simulink library "LopesDevelopmentLibrary"  (R2015b)
settings: Solver=ode45  StartTime=0.0  StopTime=10.0  RelTol=1e-3
values from neighbouring files (symbols this model uses):
  d2r = @(d) d*(pi/180)    [LopesDevelopmentLibrary_LoadParameters.m]
  ts = LopesParams.ts    [LopesDevelopmentLibrary_LoadParameters.m]
undefined symbols (not defined in the file or in its folder): anyParameterChanged, DiscIntNeverNeededParam, gcbh, LHF, LKF, LopesParams, macaddr, mxpcnetworkconfig, mxpcrtudprx, mxpcrtudptx, patientParametersChanged, port, PX, PZ, RHF, RKF, SelectorLOPESInSize, StrideTime_s, Time
undefined symbols (not defined in the file): LopesParamsSendDataArrayLen
libraries: LopesDevelopmentLibrary x288, simulink x98, dspmtrx3 x47, xpciplib x6, xpcnetworkbufferlib x5, dspsigops x4, dspstat3 x3, xpcethernetlib x2, visionstatistics x2, xpcseriallib x2, nmc x1, simulink_extras x1
(part 8 of 12)

== system LopesDevelopmentLibrary/BlocksForInternalUse/LLC Communication/UDP_Blocks/Receive_RT_2015b ==
  Buffer 1 : xpcnetworkbufferlib/Manage   ChainSize=1  BufferSize=0  Threshold=0
  Extract 1 : xpcnetworkbufferlib/Extract   PacketSize=Receive3
  Terminator : Terminator
  UDP Consume 1 : xpciplib/UDP Consume   Group=udpID  VectorSize=0  SampleTime=Receive4
  UDP Rx 1 : xpciplib/UDP Rx   Priority=5  Group=udpID  sip=Any  SourceAddress=Receive1  lup=Specify  LocalPort=Receive2  SampleTime=Receive4
  Out1 : Outport  OutDataTypeStr=uint8
  Out2 : Outport  Port=2  OutDataTypeStr=double
  wires:
  UDP Consume 1/2 -> Terminator/1
  UDP Consume 1/1 -> Extract 1/1
  UDP Rx 1/1 -> Buffer 1/1
  Buffer 1/1 -> UDP Consume 1/1
  Extract 1/1 -> Out1/1
  Extract 1/2 -> Out2/1

== system LopesDevelopmentLibrary/BlocksForInternalUse/LLC Communication/UDP_Blocks/Send_RT_2012b ==
  In1 : Inport  OutDataTypeStr=uint8
  In2 : Inport  Port=2  OutDataTypeStr=double
  "Compose " : S-Function  FunctionName=xpcnbcompose  SFunctionDeploymentMode=off  EnableBusSupport=off  mask(xpcnbcompose){}
      mask help: Network Buffer Compose
      mask init:
      | mxpcnbcompose(2);
      mask Help: helpview(fullfile(docroot, 'mapfiles', 'xpc.map'), 'NB_Compose')
      mask Display: disp('NB Compose\n');port_label('input', 2, 'length');
  "UDP Produce " : S-Function  Priority=5  FunctionName=xpcudpproduce  Parameters=Group, SrcIp, sip, DstIp, dip, LocPort, lup, RemPort, rup, SampleTime  SFunctionDeploymentMode=off  EnableBusSupport=off  mask(udpproduce){Group=0, sip=Auto, SrcIp=0.0.0.0, dip=Specify, DstIp=Send1, rup=Specify, RemPort=Send2, lup=Auto, LocPort=Send3, SampleTime=Send4}
      mask prompts: Group "IP Group"; sip "Source IP Address"; SrcIp "Source IP Address"; dip "Destination IP Address"; DstIp "IP address to send to (255.255.255.255 for broadcast):"; rup "Remote UDP Port"; RemPort "Remote IP port to send to:"; lup "Local UDP Port"; LocPort "Use the following local IP port (-1 for automatic assignment):"; SampleTime "Sample time:"
      mask help: UDP Produce
      mask init:
      | if LocPort == -1
      |     lup = 3;
      | end
      | 
      | SrcIp = ipaddr(SrcIp);
      | DstIp = ipaddr(DstIp);
      mask Help: helpview(fullfile(docroot, 'mapfiles', 'xpc.map'), 'RT_UDP_PRODUCE')
      mask TypeOptions sip: Specify | Port | Auto
      mask TypeOptions dip: Specify | Port
      mask TypeOptions rup: Specify | Port
      mask TypeOptions lup: Specify | Port | Auto
      mask Display: disp('UDP Produce');
  "UDP Tx " : xpciplib/UDP Tx   Priority=5  Group=0  TTL=-1  ToS=-1  SampleTime=Send4
  wires:
  "UDP Produce "/1 -> "UDP Tx "/1
  "Compose "/1 -> "UDP Produce "/1
  In1/1 -> "Compose "/1
  In2/1 -> "Compose "/2

== system LopesDevelopmentLibrary/BlocksForInternalUse/LLC Communication/UDP_Blocks/Send_RT_2014b ==
  In1 : Inport  OutDataTypeStr=uint8
  In2 : Inport  Port=2  OutDataTypeStr=double
  "Compose " : S-Function  FunctionName=xpcnbcompose  SFunctionDeploymentMode=off  EnableBusSupport=off  mask(xpcnbcompose){}
      mask help: Network Buffer Compose
      mask init:
      | mxpcnbcompose(2);
      mask Help: helpview(fullfile(docroot, 'mapfiles', 'xpc.map'), 'NB_Compose')
      mask Display: disp('NB Compose\n');port_label('input', 2, 'length');
  "UDP Produce " : S-Function  Priority=5  FunctionName=xpcudpproduce  Parameters=Group, SrcIp, sip, DstIp, dip, LocPort, lup, RemPort, rup, SampleTime  SFunctionDeploymentMode=off  EnableBusSupport=off  mask(udpproduce){Group=udpID, sip=Auto, SrcIp=0.0.0.0, dip=Specify, DstIp=Send1, rup=Specify, RemPort=Send2, lup=Auto, LocPort=Send3, SampleTime=Send4}
      mask prompts: Group "IP Group"; sip "Source IP Address"; SrcIp "Source IP Address"; dip "Destination IP Address"; DstIp "IP address to send to (255.255.255.255 for broadcast):"; rup "Remote UDP Port"; RemPort "Remote IP port to send to:"; lup "Local UDP Port"; LocPort "Use the following local IP port (-1 for automatic assignment):"; SampleTime "Sample time:"
      mask help: UDP Produce
      mask init:
      | if LocPort == -1
      |     lup = 3;
      | else
      |     lup = 1;
      | end
      | 
      | SrcIp = ipaddr(SrcIp);
      | DstIp = ipaddr(DstIp);
      mask Help: helpview(fullfile(docroot, 'mapfiles', 'xpc.map'), 'RT_UDP_PRODUCE')
      mask TypeOptions sip: Specify | Port | Auto
      mask TypeOptions dip: Specify | Port
      mask TypeOptions rup: Specify | Port
      mask TypeOptions lup: Specify | Port | Auto
      mask Display: disp('UDP Produce');
  "UDP Tx " : xpciplib/UDP Tx   Priority=5  Group=udpID  TTL=-1  ToS=-1  SampleTime=Send4
  wires:
  "UDP Produce "/1 -> "UDP Tx "/1
  "Compose "/1 -> "UDP Produce "/1
  In1/1 -> "Compose "/1
  In2/1 -> "Compose "/2

== system LopesDevelopmentLibrary/BlocksForInternalUse/LLC Communication/UDP_Blocks/Send_RT_2015b ==
  In1 : Inport  OutDataTypeStr=uint8
  In2 : Inport  Port=2  OutDataTypeStr=double
  "Compose " : xpcnetworkbufferlib/Compose 
  "UDP Produce " : xpciplib/UDP Produce   Priority=5  Group=udpID  sip=Auto  SrcIp=0.0.0.0  dip=Specify  DstIp=Send1  rup=Specify  RemPort=Send2  lup=Auto  LocPort=Send3  SampleTime=Send4
  "UDP Tx " : xpciplib/UDP Tx   Priority=5  Group=udpID  TTL=-1  ToS=-1  SampleTime=Send4
  wires:
  "UDP Produce "/1 -> "UDP Tx "/1
  "Compose "/1 -> "UDP Produce "/1
  In1/1 -> "Compose "/1
  In2/1 -> "Compose "/2

== system LopesDevelopmentLibrary/GaitGeneration/CalculateBreaksCoefs/Calculate/ActuatedDOFS ==

== system LopesDevelopmentLibrary/GaitGeneration/CalculateBreaksCoefs/Calculate/GenerateFakeTime ==
  note: This block generates a 'fake time' signal: (a placeholder) and a
      | fake StrideTime. These are provided in order to be able to use block that
      | require the existence of these signals. By giving fake (i.e., wrong) values,
      | the calculations in those blocks involving these signals will be wrong, but these
      | calculations are never used, so this does not matter.
  Bus Creator13 : BusCreator  Inputs=2
  FakeBreaksTime : Constant  Value=[0,100]
  FakeCoefsTime : Constant  Value=[0,0,0;0,0,0]
  FakeStrideTime1 : Constant
  FakeStrideTime_s : Outport
  FakeTime : Outport  Port=2
  wires:
  FakeCoefsTime/1 -> Bus Creator13/2  "coefs"
  FakeBreaksTime/1 -> Bus Creator13/1  "breaks"
  Bus Creator13/1 -> FakeTime/1  "Time"
  FakeStrideTime1/1 -> FakeStrideTime_s/1

== system LopesDevelopmentLibrary/GaitGeneration/CalculateBreaksCoefs/Calculate/LeftAnkleZ1 ==
  note: Maximum of 15 cm extra circumduction
  parameters : Inport
  WeightShift_StepWidth_pct : Inport  Port=2
  Circumduction_CircumductionLeft_pct : Inport  Port=3
  AddToMatrixElement : LopesDevelopmentLibrary/Various/AddToMatrixElement  row=3  col=2  minimum=-inf  maximum=inf
  AssignMatrixElement : LopesDevelopmentLibrary/Various/AssignMatrixElement  row=3  col=2  minimum=-inf  maximum=inf
  Bias : Bias  Bias=1
  CircumductionGain : Gain  Gain=0.01*(-0.15)
  Gain2 : Gain  Gain=0.01
  K1toK3 : dspmtrx3/Submatrix  RowSpan=All rows  RowStartMode=Index  RowStartIndex=row  RowEndMode=Index  RowEndIndex=1  ColSpan=One column  ColStartMode=Index  ColStartIndex=2  ColEndMode=Last  ColEndIndex=1
  MinMax : MinMax
  MultiplyMatrixElement : LopesDevelopmentLibrary/Various/MultiplyMatrixElement  row=1  col=2  minimum=-inf  maximum=inf
  MultiplyMatrixElement1 : LopesDevelopmentLibrary/Various/MultiplyMatrixElement  row=2  col=2  minimum=-inf  maximum=inf
  RegressionData : Constant  Value=LopesParams.GaitData.LAnkleZ
  RegressionData2KeyEvents : LopesDevelopmentLibrary/BlocksForInternalUse/GaitGeneration/RegressionData2KeyEvents
  KeyEvents : Outport
  wires:
  RegressionData2KeyEvents/1 -> MultiplyMatrixElement/1
  RegressionData/1 -> RegressionData2KeyEvents/1
  parameters/1 -> RegressionData2KeyEvents/2
  WeightShift_StepWidth_pct/1 -> Gain2/1
  Gain2/1 -> Bias/1
  Bias/1 -> MultiplyMatrixElement/2, MultiplyMatrixElement1/2
  AddToMatrixElement/1 -> KeyEvents/1
  MultiplyMatrixElement/1 -> MultiplyMatrixElement1/1
  MultiplyMatrixElement1/1 -> K1toK3/1, AssignMatrixElement/1
  K1toK3/1 -> MinMax/1
  MinMax/1 -> AssignMatrixElement/2
  AssignMatrixElement/1 -> AddToMatrixElement/1
  Circumduction_CircumductionLeft_pct/1 -> CircumductionGain/1
  CircumductionGain/1 -> AddToMatrixElement/2

== system LopesDevelopmentLibrary/GaitGeneration/CalculateBreaksCoefs/Calculate/LeftHipFlexion1 ==
  parameters : Inport
  HipExtensionOffset_pct : Inport  Port=2
  Steplength_Length_pct : Inport  Port=3
  SteplengthOtherLeg_Length_pct : Inport  Port=4
  StepHeight_KneeFlexion_pct : Inport  Port=5
  AddToMatrixColumn : LopesDevelopmentLibrary/Various/AddToMatrixColumn  col=2  minimum=-inf  maximum=inf
  Bias : Bias  Bias=100
  Bias1 : Bias  Bias=100
  Gain1 : Gain  Gain=1/100
  Gain2 : Gain  Gain=1/100
  Gain3 : Gain  Gain=0.01* d2r(2.5)
  Gain4 : Gain  Gain=0.01* d2r(5)
  GainHipExtensionOffset : Gain  Gain=-0.01* d2r(10)
  KneeFlexionStepheight : LopesDevelopmentLibrary/Various/AddToMatrixElement  row=5  col=2  minimum=0  maximum=d2r(90)
  KneeFlexionStepheight1 : LopesDevelopmentLibrary/Various/AddToMatrixElement  row=6  col=2  minimum=0  maximum=d2r(90)
  MultiplyMatrixElement : LopesDevelopmentLibrary/Various/MultiplyMatrixElement  row=6  col=2  minimum=-inf  maximum=inf
  MultiplyMatrixElement1 : LopesDevelopmentLibrary/Various/MultiplyMatrixElement  row=4  col=2  minimum=-inf  maximum=inf
  MultiplyMatrixElement2 : LopesDevelopmentLibrary/Various/MultiplyMatrixElement  row=1  col=2  minimum=-inf  maximum=inf
  MultiplyMatrixElement3 : LopesDevelopmentLibrary/Various/MultiplyMatrixElement  row=2  col=2  minimum=-inf  maximum=inf
  RatioFlexionExtension : Gain
  RegressionData : Constant  Value=LopesParams.GaitData.LHF
  RegressionData2KeyEvents : LopesDevelopmentLibrary/BlocksForInternalUse/GaitGeneration/RegressionData2KeyEvents
  KeyEvents : Outport
  wires:
  MultiplyMatrixElement1/1 -> KeyEvents/1
  AddToMatrixColumn/1 -> MultiplyMatrixElement/1
  Gain2/1 -> MultiplyMatrixElement1/2
  Steplength_Length_pct/1 -> Bias/1
  Bias/1 -> Gain1/1
  Gain1/1 -> MultiplyMatrixElement3/2, MultiplyMatrixElement2/2, MultiplyMatrixElement/2
  Bias1/1 -> Gain2/1
  SteplengthOtherLeg_Length_pct/1 -> RatioFlexionExtension/1
  RegressionData/1 -> RegressionData2KeyEvents/1
  parameters/1 -> RegressionData2KeyEvents/2
  KneeFlexionStepheight/1 -> KneeFlexionStepheight1/1
  RegressionData2KeyEvents/1 -> KneeFlexionStepheight/1
  Gain3/1 -> KneeFlexionStepheight/2
  Gain4/1 -> KneeFlexionStepheight1/2
  StepHeight_KneeFlexion_pct/1 -> Gain4/1, Gain3/1
  HipExtensionOffset_pct/1 -> GainHipExtensionOffset/1
  KneeFlexionStepheight1/1 -> AddToMatrixColumn/1
  GainHipExtensionOffset/1 -> AddToMatrixColumn/2
  RatioFlexionExtension/1 -> Bias1/1
  MultiplyMatrixElement/1 -> MultiplyMatrixElement2/1
  MultiplyMatrixElement2/1 -> MultiplyMatrixElement3/1
  MultiplyMatrixElement3/1 -> MultiplyMatrixElement1/1

== system LopesDevelopmentLibrary/GaitGeneration/CalculateBreaksCoefs/Calculate/LeftKneeFlexion1 ==
  parameters : Inport
  StepHeight_KneeFlexion_pct : Inport  Port=2
  Prepositioning_KneeFlexion_pct : Inport  Port=3
  StabilityStance_Kneeflexion_pct : Inport  Port=4
  StepLength_pct : Inport  Port=5
  Constant : Constant  Value=-inf
  Gain1 : Gain  Gain=0.01* d2r(5)
  Gain2 : Gain  Gain=0.01* d2r(10)
  Gain3 : Gain  Gain=0.01* d2r(5)
  Gain4 : Gain  Gain=0.01* d2r(20)
  Gain5 : Gain  Gain=-0.01/3
  KneeFlexionPrepositioning : LopesDevelopmentLibrary/Various/AddToMatrixElement  row=1  col=2  minimum=0  maximum=d2r(90)
  KneefFlexionStepheigh : LopesDevelopmentLibrary/Various/AddToMatrixElement  row=5  col=2  minimum=0  maximum=d2r(90)
  KneefFlexionStepheigh1 : LopesDevelopmentLibrary/Various/AddToMatrixElement  row=6  col=2  minimum=0  maximum=d2r(90)
  KneeflexionStance : LopesDevelopmentLibrary/Various/AddToMatrixElement  row=2  col=2  minimum=0  maximum=d2r(90)
  RatioKey6toKey1 : Gain  Gain=1/2
  RegressionData : Constant  Value=LopesParams.GaitData.LKF
  RegressionData2KeyEvents : LopesDevelopmentLibrary/BlocksForInternalUse/GaitGeneration/RegressionData2KeyEvents
  Saturation : Saturate  UpperLimit=0  LowerLimit=-inf
  Saturation Dynamic : simulink/Discontinuities/Saturation Dynamic  OutMin=[]  OutMax=[]  OutDataTypeStr=Inherit: Same as second input  OutDataType=fixdt(1, 16)  OutScaling=2^-10  DoSatur=off
  SelectorK1 : Selector  NumberOfDimensions=2  InputPortWidth=3  IndexOptions=Index vector (dialog),Index vector (dialog)  Indices=1,2  OutputSizes=1,1
  SelectorK2 : Selector  NumberOfDimensions=2  InputPortWidth=3  IndexOptions=Index vector (dialog),Index vector (dialog)  Indices=2,2  OutputSizes=1,1
  Steplength1 : LopesDevelopmentLibrary/Various/AddToMatrixElement  row=1  col=2  minimum=0  maximum=d2r(90)
  Steplength2 : LopesDevelopmentLibrary/Various/AddToMatrixElement  row=6  col=2  minimum=0  maximum=d2r(90)
  Sum : Sum  Inputs=++|
  Sum1 : Sum  Inputs=-+|
  KeyEvents : Outport
  wires:
  Gain1/1 -> KneeFlexionPrepositioning/2
  StabilityStance_Kneeflexion_pct/1 -> Gain3/1
  Prepositioning_KneeFlexion_pct/1 -> Gain1/1
  RegressionData/1 -> RegressionData2KeyEvents/1
  parameters/1 -> RegressionData2KeyEvents/2
  KneeFlexionPrepositioning/1 -> KneeflexionStance/1
  RegressionData2KeyEvents/1 -> KneefFlexionStepheigh/1
  KneefFlexionStepheigh/1 -> KneefFlexionStepheigh1/1
  StepHeight_KneeFlexion_pct/1 -> Gain4/1, Gain2/1
  Gain2/1 -> KneefFlexionStepheigh/2
  Gain3/1 -> KneeflexionStance/2
  KneefFlexionStepheigh1/1 -> KneeFlexionPrepositioning/1
  Gain4/1 -> KneefFlexionStepheigh1/2
  StepLength_pct/1 -> Saturation/1
  Steplength1/1 -> Steplength2/1
  Steplength2/1 -> KeyEvents/1
  KneeflexionStance/1 -> SelectorK1/1, SelectorK2/1, Steplength1/1
  RatioKey6toKey1/1 -> Steplength2/2
  SelectorK2/1 -> Saturation Dynamic/1
  Constant/1 -> Saturation Dynamic/3
  SelectorK1/1 -> Sum1/1, Sum/1
  Gain5/1 -> Sum/2
  Sum/1 -> Saturation Dynamic/2
  Sum1/1 -> RatioKey6toKey1/1, Steplength1/2
  Saturation Dynamic/1 -> Sum1/2
  Saturation/1 -> Gain5/1

== system LopesDevelopmentLibrary/GaitGeneration/CalculateBreaksCoefs/Calculate/PelvisAxialRotation1 ==
  parameters : Inport
  RegressionData : Constant  Value=LopesParams.GaitData.PAX
  RegressionData2KeyEvents : LopesDevelopmentLibrary/BlocksForInternalUse/GaitGeneration/RegressionData2KeyEvents
  KeyEvents : Outport
  wires:
  parameters/1 -> RegressionData2KeyEvents/2
  RegressionData/1 -> RegressionData2KeyEvents/1
  RegressionData2KeyEvents/1 -> KeyEvents/1

== system LopesDevelopmentLibrary/GaitGeneration/CalculateBreaksCoefs/Calculate/PelvisObliquity1 ==
  parameters : Inport
  RegressionData : Constant  Value=LopesParams.GaitData.POB
  RegressionData2KeyEvents : LopesDevelopmentLibrary/BlocksForInternalUse/GaitGeneration/RegressionData2KeyEvents
  KeyEvents : Outport
  wires:
  RegressionData2KeyEvents/1 -> KeyEvents/1
  RegressionData/1 -> RegressionData2KeyEvents/1
  parameters/1 -> RegressionData2KeyEvents/2

== system LopesDevelopmentLibrary/GaitGeneration/CalculateBreaksCoefs/Calculate/PelvisTX1 ==
  parameters : Inport
  RegressionData : Constant  Value=LopesParams.GaitData.PX
  RegressionData2KeyEvents : LopesDevelopmentLibrary/BlocksForInternalUse/GaitGeneration/RegressionData2KeyEvents
  KeyEvents : Outport
  wires:
  RegressionData2KeyEvents/1 -> KeyEvents/1
  RegressionData/1 -> RegressionData2KeyEvents/1
  parameters/1 -> RegressionData2KeyEvents/2

== system LopesDevelopmentLibrary/GaitGeneration/CalculateBreaksCoefs/Calculate/PelvisTY1 ==
  parameters : Inport
  RegressionData : Constant  Value=LopesParams.GaitData.PY
  RegressionData2KeyEvents : LopesDevelopmentLibrary/BlocksForInternalUse/GaitGeneration/RegressionData2KeyEvents
  KeyEvents : Outport
  wires:
  RegressionData2KeyEvents/1 -> KeyEvents/1
  RegressionData/1 -> RegressionData2KeyEvents/1
  parameters/1 -> RegressionData2KeyEvents/2

== system LopesDevelopmentLibrary/GaitGeneration/CalculateBreaksCoefs/Calculate/PelvisTZ1 ==
  Parameters : Inport
  WeightShift_AmplitudeLeft_pct : Inport  Port=2
  WeightShift_AmplitudeRight_pct : Inport  Port=3
  WeightShift_Timing_pct : Inport  Port=4
  WeightShift_DurationLeft_pct : Inport  Port=5
  WeightShift_DurationRight_pct : Inport  Port=6
  AdjustAmplitude : Subsystem
  AdjustDurationLeft : Subsystem  mask{keyEventsToAffect=[1,2], keyEventBeforeAffected=6}
      mask prompts: keyEventsToAffect "Affect which key events (give two)"; keyEventBeforeAffected "Index of key event just before affected ones"
  AdjustDurationRight : Subsystem  mask{keyEventsToAffect=[4,5], keyEventBeforeAffected=3}
      mask prompts: keyEventsToAffect "Affect which key events (give two)"; keyEventBeforeAffected "Index of key event just before affected ones"
  AdjustTiming : LopesDevelopmentLibrary/Various/AddToMatrixColumn  col=1  minimum=-inf  maximum=inf
  Bias : Bias  Bias=1
  Bias1 : Bias  Bias=1
  Gain1 : Gain  Gain=0.01
  Gain2 : Gain  Gain=0.01
  RegressionData : Constant  Value=LopesParams.GaitData.PZ
  RegressionData2KeyEvents : LopesDevelopmentLibrary/BlocksForInternalUse/GaitGeneration/RegressionData2KeyEvents
  Saturation : Saturate  UpperLimit=2  LowerLimit=0
  Saturation1 : Saturate  UpperLimit=2  LowerLimit=0
  KeyEvents : Outport
  wires:
  Bias/1 -> Saturation/1
  RegressionData/1 -> RegressionData2KeyEvents/1
  WeightShift_Timing_pct/1 -> AdjustTiming/2
  WeightShift_DurationLeft_pct/1 -> AdjustDurationLeft/2(V)
  WeightShift_AmplitudeLeft_pct/1 -> Gain2/1
  AdjustAmplitude/1(Y) -> AdjustDurationLeft/1(M)
  AdjustTiming/1 -> KeyEvents/1
  Gain2/1 -> Bias/1
  Parameters/1 -> RegressionData2KeyEvents/2
  RegressionData2KeyEvents/1 -> AdjustAmplitude/1(M)
  Saturation/1 -> AdjustAmplitude/2(V_left)
  AdjustDurationRight/1(Y) -> AdjustTiming/1
  AdjustDurationLeft/1(Y) -> AdjustDurationRight/1(M)
  WeightShift_DurationRight_pct/1 -> AdjustDurationRight/2(V)
  Bias1/1 -> Saturation1/1
  Gain1/1 -> Bias1/1
  WeightShift_AmplitudeRight_pct/1 -> Gain1/1
  Saturation1/1 -> AdjustAmplitude/3(V_right)

== system LopesDevelopmentLibrary/GaitGeneration/CalculateBreaksCoefs/Calculate/RightAnkleZ1 ==
  note: Maximum of 15 cm extra circumduction
  parameters : Inport
  WeightShift_StepWidth_pct : Inport  Port=2
  Circumduction_CircumductionRight_pct : Inport  Port=3
  AddToMatrixElement : LopesDevelopmentLibrary/Various/AddToMatrixElement  row=3  col=2  minimum=-inf  maximum=inf
  AssignMatrixElement : LopesDevelopmentLibrary/Various/AssignMatrixElement  row=3  col=2  minimum=-inf  maximum=inf
  Bias : Bias  Bias=1
  CircumductionGain : Gain  Gain=0.01*(0.15)
  Gain2 : Gain  Gain=0.01
  K1toK3 : dspmtrx3/Submatrix  RowSpan=All rows  RowStartMode=Index  RowStartIndex=row  RowEndMode=Index  RowEndIndex=1  ColSpan=One column  ColStartMode=Index  ColStartIndex=2  ColEndMode=Last  ColEndIndex=1
  MinMax : MinMax  Function=max
  MultiplyMatrixElement : LopesDevelopmentLibrary/Various/MultiplyMatrixElement  row=1  col=2  minimum=-inf  maximum=inf
  MultiplyMatrixElement1 : LopesDevelopmentLibrary/Various/MultiplyMatrixElement  row=2  col=2  minimum=-inf  maximum=inf
  RegressionData : Constant  Value=LopesParams.GaitData.RAnkleZ
  RegressionData2KeyEvents : LopesDevelopmentLibrary/BlocksForInternalUse/GaitGeneration/RegressionData2KeyEvents
  KeyEvents : Outport
  wires:
  CircumductionGain/1 -> AddToMatrixElement/2
  Circumduction_CircumductionRight_pct/1 -> CircumductionGain/1
  AssignMatrixElement/1 -> AddToMatrixElement/1
  MinMax/1 -> AssignMatrixElement/2
  K1toK3/1 -> MinMax/1
  MultiplyMatrixElement1/1 -> AssignMatrixElement/1, K1toK3/1
  MultiplyMatrixElement/1 -> MultiplyMatrixElement1/1
  AddToMatrixElement/1 -> KeyEvents/1
  Bias/1 -> MultiplyMatrixElement1/2, MultiplyMatrixElement/2
  Gain2/1 -> Bias/1
  WeightShift_StepWidth_pct/1 -> Gain2/1
  parameters/1 -> RegressionData2KeyEvents/2
  RegressionData/1 -> RegressionData2KeyEvents/1
  RegressionData2KeyEvents/1 -> MultiplyMatrixElement/1

== system LopesDevelopmentLibrary/GaitGeneration/CalculateBreaksCoefs/Calculate/RightHipFlexion1 ==
  parameters : Inport
  HipExtensionOffset_pct : Inport  Port=2
  Steplength_Length_pct : Inport  Port=3
  SteplengthOtherLeg_Length_pct : Inport  Port=4
  StepHeight_KneeFlexion_pct : Inport  Port=5
  AddToMatrixColumn : LopesDevelopmentLibrary/Various/AddToMatrixColumn  col=2  minimum=-inf  maximum=inf
  Bias : Bias  Bias=100
  Bias1 : Bias  Bias=100
  Gain1 : Gain  Gain=1/100
  Gain2 : Gain  Gain=1/100
  Gain3 : Gain  Gain=0.01* d2r(2.5)
  Gain4 : Gain  Gain=0.01* d2r(5)
  GainHipExtensionOffset : Gain  Gain=-0.01* d2r(10)
  KneeFlexionStepheight : LopesDevelopmentLibrary/Various/AddToMatrixElement  row=5  col=2  minimum=0  maximum=d2r(90)
  KneeFlexionStepheight1 : LopesDevelopmentLibrary/Various/AddToMatrixElement  row=6  col=2  minimum=0  maximum=d2r(90)
  MultiplyMatrixElement : LopesDevelopmentLibrary/Various/MultiplyMatrixElement  row=6  col=2  minimum=-inf  maximum=inf
  MultiplyMatrixElement1 : LopesDevelopmentLibrary/Various/MultiplyMatrixElement  row=4  col=2  minimum=-inf  maximum=inf
  MultiplyMatrixElement2 : LopesDevelopmentLibrary/Various/MultiplyMatrixElement  row=1  col=2  minimum=-inf  maximum=inf
  MultiplyMatrixElement3 : LopesDevelopmentLibrary/Various/MultiplyMatrixElement  row=2  col=2  minimum=-inf  maximum=inf
  RatioFlexionExtension : Gain
  RegressionData : Constant  Value=LopesParams.GaitData.RHF
  RegressionData2KeyEvents : LopesDevelopmentLibrary/BlocksForInternalUse/GaitGeneration/RegressionData2KeyEvents
  KeyEvents : Outport
  wires:
  MultiplyMatrixElement1/1 -> KeyEvents/1
  AddToMatrixColumn/1 -> MultiplyMatrixElement/1
  Gain2/1 -> MultiplyMatrixElement1/2
  Steplength_Length_pct/1 -> Bias/1
  Bias/1 -> Gain1/1
  Gain1/1 -> MultiplyMatrixElement3/2, MultiplyMatrixElement2/2, MultiplyMatrixElement/2
  Bias1/1 -> Gain2/1
  SteplengthOtherLeg_Length_pct/1 -> RatioFlexionExtension/1
  RegressionData/1 -> RegressionData2KeyEvents/1
  parameters/1 -> RegressionData2KeyEvents/2
  KneeFlexionStepheight/1 -> KneeFlexionStepheight1/1
  RegressionData2KeyEvents/1 -> KneeFlexionStepheight/1
  Gain3/1 -> KneeFlexionStepheight/2
  Gain4/1 -> KneeFlexionStepheight1/2
  StepHeight_KneeFlexion_pct/1 -> Gain4/1, Gain3/1
  HipExtensionOffset_pct/1 -> GainHipExtensionOffset/1
  KneeFlexionStepheight1/1 -> AddToMatrixColumn/1
  GainHipExtensionOffset/1 -> AddToMatrixColumn/2
  RatioFlexionExtension/1 -> Bias1/1
  MultiplyMatrixElement/1 -> MultiplyMatrixElement2/1
  MultiplyMatrixElement2/1 -> MultiplyMatrixElement3/1
  MultiplyMatrixElement3/1 -> MultiplyMatrixElement1/1

== system LopesDevelopmentLibrary/GaitGeneration/CalculateBreaksCoefs/Calculate/RightKneeFlexion1 ==
  parameters : Inport
  StepHeight_KneeFlexion_pct : Inport  Port=2
  Prepositioning_KneeFlexion_pct : Inport  Port=3
  StabilityStance_Kneeflexion_pct : Inport  Port=4
  StepLength_pct : Inport  Port=5
  Constant : Constant  Value=-inf
  Gain1 : Gain  Gain=0.01* d2r(5)
  Gain2 : Gain  Gain=0.01* d2r(10)
  Gain3 : Gain  Gain=0.01* d2r(5)
  Gain4 : Gain  Gain=0.01* d2r(20)
  Gain5 : Gain  Gain=-0.01/3
  KneeFlexionPrepositioning : LopesDevelopmentLibrary/Various/AddToMatrixElement  row=1  col=2  minimum=0  maximum=d2r(90)
  KneefFlexionStepheigh : LopesDevelopmentLibrary/Various/AddToMatrixElement  row=5  col=2  minimum=0  maximum=d2r(90)
  KneefFlexionStepheigh1 : LopesDevelopmentLibrary/Various/AddToMatrixElement  row=6  col=2  minimum=0  maximum=d2r(90)
  KneeflexionStance : LopesDevelopmentLibrary/Various/AddToMatrixElement  row=2  col=2  minimum=0  maximum=d2r(90)
  RatioKey6toKey1 : Gain  Gain=1/2
  RegressionData : Constant  Value=LopesParams.GaitData.RKF
  RegressionData2KeyEvents : LopesDevelopmentLibrary/BlocksForInternalUse/GaitGeneration/RegressionData2KeyEvents
  Saturation : Saturate  UpperLimit=0  LowerLimit=-inf
  Saturation Dynamic : simulink/Discontinuities/Saturation Dynamic  OutMin=[]  OutMax=[]  OutDataTypeStr=Inherit: Same as second input  OutDataType=fixdt(1, 16)  OutScaling=2^-10  DoSatur=off
  SelectorK1 : Selector  NumberOfDimensions=2  InputPortWidth=3  IndexOptions=Index vector (dialog),Index vector (dialog)  Indices=1,2  OutputSizes=1,1
  SelectorK2 : Selector  NumberOfDimensions=2  InputPortWidth=3  IndexOptions=Index vector (dialog),Index vector (dialog)  Indices=2,2  OutputSizes=1,1
  Steplength1 : LopesDevelopmentLibrary/Various/AddToMatrixElement  row=1  col=2  minimum=0  maximum=d2r(90)
  Steplength2 : LopesDevelopmentLibrary/Various/AddToMatrixElement  row=6  col=2  minimum=0  maximum=d2r(90)
  Sum : Sum  Inputs=++|
  Sum1 : Sum  Inputs=-+|
  KeyEvents : Outport
  wires:
  Gain4/1 -> KneefFlexionStepheigh1/2
  KneefFlexionStepheigh1/1 -> KneeFlexionPrepositioning/1
  Gain3/1 -> KneeflexionStance/2
  Gain2/1 -> KneefFlexionStepheigh/2
  StepHeight_KneeFlexion_pct/1 -> Gain2/1, Gain4/1
  KneefFlexionStepheigh/1 -> KneefFlexionStepheigh1/1
  RegressionData2KeyEvents/1 -> KneefFlexionStepheigh/1
  KneeFlexionPrepositioning/1 -> KneeflexionStance/1
  parameters/1 -> RegressionData2KeyEvents/2
  RegressionData/1 -> RegressionData2KeyEvents/1
  Prepositioning_KneeFlexion_pct/1 -> Gain1/1
  StabilityStance_Kneeflexion_pct/1 -> Gain3/1
  Gain1/1 -> KneeFlexionPrepositioning/2
  StepLength_pct/1 -> Saturation/1
  Steplength1/1 -> Steplength2/1
  RatioKey6toKey1/1 -> Steplength2/2
  SelectorK2/1 -> Saturation Dynamic/1
  Constant/1 -> Saturation Dynamic/3
  SelectorK1/1 -> Sum1/1, Sum/1
  Gain5/1 -> Sum/2
  Sum/1 -> Saturation Dynamic/2
  Sum1/1 -> RatioKey6toKey1/1, Steplength1/2
  Saturation Dynamic/1 -> Sum1/2
  Saturation/1 -> Gain5/1
  Steplength2/1 -> KeyEvents/1
  KneeflexionStance/1 -> SelectorK1/1, SelectorK2/1, Steplength1/1

== system LopesDevelopmentLibrary/GaitGeneration/CalculateBreaksCoefs/Calculate/Time1 ==
  note: v = strideLengh * nStridesPerSecond
      |                   = strideLength / nSecondsPerStride
      | strideTime = nSecondsPerStride = strideLength / v
  note: The key event matrix is generated here; it consists
      | of two rows (ie, a key event at 0% and one at 100%),
      | and the start time (=0) and end time. We need to
      | calculate the slope (in s/%) as well to get a straight line.
  WalkingVelocity_m_s : Inport
  BreaksCoefsBus : Inport  Port=2
  Parameters : Inport  Port=3
  CalculateStrideLength : Subsystem
  Constant : Constant  Value=[0,0,nan; 100,nan,nan]
  Gain : Gain  Gain=0.01
  Mux : Mux  Inputs=2
  Overwrite Values : dspmtrx3/Overwrite Values  OverWriteDiag=Submatrix  valFrom2ndIP=Second input port  ConstValue=0  RowSpan=One row  RowStartMode=Index  RowStartIndex=2  RowEndMode=Last  RowEndIndex=1  ColSpan=One column  ColStartMode=Index  ColStartIndex=2  ColEndMode=Last  ColEndIndex=1  DiagSpan=Range of elements  DiagStartMode=Index  DiagStartIndex=2  DiagEndMode=Index  DiagEndIndex=4
  Overwrite Values1 : dspmtrx3/Overwrite Values  OverWriteDiag=Submatrix  valFrom2ndIP=Second input port  ConstValue=0  RowSpan=All rows  RowStartMode=Index  RowStartIndex=2  RowEndMode=Last  RowEndIndex=1  ColSpan=One column  ColStartMode=Last  ColStartIndex=2  ColEndMode=Last  ColEndIndex=1  DiagSpan=Range of elements  DiagStartMode=Index  DiagStartIndex=2  DiagEndMode=Index  DiagEndIndex=4
  SafeDivide : LopesDevelopmentLibrary/Various/SafeDivide  SystemSampleTime=-1
  KeyEvents : Outport
  StrideTime_s : Outport  Port=2
  wires:
  Mux/1 -> Overwrite Values1/2
  Overwrite Values/1 -> Overwrite Values1/1
  Gain/1 -> Mux/2, Mux/1  "slope"
  Constant/1 -> Overwrite Values/1
  SafeDivide/1 -> StrideTime_s/1, Gain/1, Overwrite Values/2  "StrideTime"
  Overwrite Values1/1 -> KeyEvents/1
  BreaksCoefsBus/1 -> CalculateStrideLength/1(BreaksCoefsBus)
  Parameters/1 -> CalculateStrideLength/2(Parameters)
  WalkingVelocity_m_s/1 -> SafeDivide/2
  CalculateStrideLength/1(StrideLength) -> SafeDivide/1

== system LopesDevelopmentLibrary/GaitGeneration/CalculateBreaksCoefs/Calculate/Unactuated DOFS ==

== system LopesDevelopmentLibrary/GaitGeneration/PhaseEstimatorAoyagi/EstimatePhaseDirectlyAoyagi/CalculateFullReferenceTrajectory ==
  BreaksCoefs : Inport
  xx : Inport  Port=2
  Enable : EnablePort
  Bus Selector2 : BusSelector  OutputSignals=LHF,LKF,RHF,RKF,StrideTime_s
  Divide{,1,3..4} (4 alike) : Product  Inputs=*/
  Gain : Gain  Gain=0.01
  Terminator{,1,3..4} (4 alike) : Terminator
  ppval_bus_LHF : LopesDevelopmentLibrary/BlocksForInternalUse/GaitGeneration/ppval_bus
  ppval_bus_LKF : LopesDevelopmentLibrary/BlocksForInternalUse/GaitGeneration/ppval_bus
  ppval_bus_RHF : LopesDevelopmentLibrary/BlocksForInternalUse/GaitGeneration/ppval_bus
  ppval_bus_RKF : LopesDevelopmentLibrary/BlocksForInternalUse/GaitGeneration/ppval_bus
  LHF_yy : Outport
  LKF_yy : Outport  Port=2
  RHF_yy : Outport  Port=3
  RKF_yy : Outport  Port=4
  LHF_dydt : Outport  Port=5
  LKF_dydt : Outport  Port=6
  RHF_dydt : Outport  Port=7
  RKF_dydt : Outport  Port=8
  wires:
  ppval_bus_LKF/1 -> LKF_yy/1
  ppval_bus_LHF/1 -> LHF_yy/1
  Bus Selector2/5 -> Gain/1  "<StrideTime_s>"
  Bus Selector2/4 -> ppval_bus_RKF/2  "<RKF>"
  Bus Selector2/3 -> ppval_bus_RHF/2  "<RHF>"
  Bus Selector2/2 -> ppval_bus_LKF/2  "<LKF>"
  Bus Selector2/1 -> ppval_bus_LHF/2  "<LHF>"
  ppval_bus_RHF/1 -> RHF_yy/1
  ppval_bus_RKF/1 -> RKF_yy/1
  ppval_bus_LHF/2 -> Divide/1
  ppval_bus_LKF/2 -> Divide1/1
  ppval_bus_RHF/2 -> Divide3/1
  ppval_bus_RKF/2 -> Divide4/1
  Gain/1 -> Divide4/2, Divide3/2, Divide1/2, Divide/2  "dtdx"
  Divide/1 -> LHF_dydt/1
  Divide1/1 -> LKF_dydt/1
  Divide3/1 -> RHF_dydt/1
  Divide4/1 -> RKF_dydt/1
  ppval_bus_LHF/3 -> Terminator/1
  ppval_bus_RKF/3 -> Terminator4/1
  ppval_bus_LKF/3 -> Terminator1/1
  ppval_bus_RHF/3 -> Terminator3/1
  BreaksCoefs/1 -> Bus Selector2/1
  xx/1 -> ppval_bus_LHF/1, ppval_bus_LKF/1, ppval_bus_RKF/1, ppval_bus_RHF/1

== system LopesDevelopmentLibrary/GaitGeneration/PhaseEstimatorAoyagi/PhaseFilterAoyagi/Wrap_Min50_Plus50 ==
  note: Wraps the input phase such
      | that the output is always
      | in the range -50<=out<50
      | (even if input is negative).
  In : Inport
  Bias : Bias  Bias=50
  Bias1 : Bias  Bias=-50
  Constant1 : Constant  Value=100
  ShiftedPhase1 : Math  Operator=mod  SaturateOnIntegerOverflow=on
  Out : Outport
  wires:
  ShiftedPhase1/1 -> Bias1/1
  In/1 -> Bias/1
  Constant1/1 -> ShiftedPhase1/2
  Bias/1 -> ShiftedPhase1/1
  Bias1/1 -> Out/1

== system LopesDevelopmentLibrary/GaitGeneration/PhaseEstimatorAoyagi_wPI/EstimatePhaseDirectlyAoyagi/CalculateFullReferenceTrajectory ==
  BreaksCoefs : Inport
  xx : Inport  Port=2
  Enable : EnablePort
  Bus Selector2 : BusSelector  OutputSignals=LHF,LKF,RHF,RKF,StrideTime_s
  Divide{,1,3..4} (4 alike) : Product  Inputs=*/
  Gain : Gain  Gain=0.01
  Terminator{,1,3..4} (4 alike) : Terminator
  ppval_bus_LHF : LopesDevelopmentLibrary/BlocksForInternalUse/GaitGeneration/ppval_bus
  ppval_bus_LKF : LopesDevelopmentLibrary/BlocksForInternalUse/GaitGeneration/ppval_bus
  ppval_bus_RHF : LopesDevelopmentLibrary/BlocksForInternalUse/GaitGeneration/ppval_bus
  ppval_bus_RKF : LopesDevelopmentLibrary/BlocksForInternalUse/GaitGeneration/ppval_bus
  LHF_yy : Outport
  LKF_yy : Outport  Port=2
  RHF_yy : Outport  Port=3
  RKF_yy : Outport  Port=4
  LHF_dydt : Outport  Port=5
  LKF_dydt : Outport  Port=6
  RHF_dydt : Outport  Port=7
  RKF_dydt : Outport  Port=8
  wires:
  ppval_bus_LKF/1 -> LKF_yy/1
  ppval_bus_LHF/1 -> LHF_yy/1
  Bus Selector2/5 -> Gain/1  "<StrideTime_s>"
  Bus Selector2/4 -> ppval_bus_RKF/2  "<RKF>"
  Bus Selector2/3 -> ppval_bus_RHF/2  "<RHF>"
  Bus Selector2/2 -> ppval_bus_LKF/2  "<LKF>"
  Bus Selector2/1 -> ppval_bus_LHF/2  "<LHF>"
  ppval_bus_RHF/1 -> RHF_yy/1
  ppval_bus_RKF/1 -> RKF_yy/1
  ppval_bus_LHF/2 -> Divide/1
  ppval_bus_LKF/2 -> Divide1/1
  ppval_bus_RHF/2 -> Divide3/1
  ppval_bus_RKF/2 -> Divide4/1
  Gain/1 -> Divide4/2, Divide3/2, Divide1/2, Divide/2  "dtdx"
  Divide/1 -> LHF_dydt/1
  Divide1/1 -> LKF_dydt/1
  Divide3/1 -> RHF_dydt/1
  Divide4/1 -> RKF_dydt/1
  ppval_bus_LHF/3 -> Terminator/1
  ppval_bus_RKF/3 -> Terminator4/1
  ppval_bus_LKF/3 -> Terminator1/1
  ppval_bus_RHF/3 -> Terminator3/1
  BreaksCoefs/1 -> Bus Selector2/1
  xx/1 -> ppval_bus_LHF/1, ppval_bus_LKF/1, ppval_bus_RKF/1, ppval_bus_RHF/1

== system LopesDevelopmentLibrary/GaitGeneration/PhaseEstimatorAoyagi_wPI/PhaseFilterAoyagi/Wrap_Min50_Plus50 ==
  note: Wraps the input phase such
      | that the output is always
      | in the range -50<=out<50
      | (even if input is negative).
  In : Inport
  Bias : Bias  Bias=50
  Bias1 : Bias  Bias=-50
  Constant1 : Constant  Value=100
  ShiftedPhase1 : Math  Operator=mod  SaturateOnIntegerOverflow=on
  Out : Outport
  wires:
  ShiftedPhase1/1 -> Bias1/1
  In/1 -> Bias/1
  Constant1/1 -> ShiftedPhase1/2
  Bias/1 -> ShiftedPhase1/1
  Bias1/1 -> Out/1

== system LopesDevelopmentLibrary/GaitGenerationExtra/CalculateBreaksCoefs/Calculate/ActuatedDOFS ==

== system LopesDevelopmentLibrary/GaitGenerationExtra/CalculateBreaksCoefs/Calculate/GenerateFakeTime ==
  note: This block generates a 'fake time' signal: (a placeholder) and a
      | fake StrideTime. These are provided in order to be able to use block that
      | require the existence of these signals. By giving fake (i.e., wrong) values,
      | the calculations in those blocks involving these signals will be wrong, but these
      | calculations are never used, so this does not matter.
  Bus Creator13 : BusCreator  Inputs=2
  FakeBreaksTime : Constant  Value=[0,100]
  FakeCoefsTime : Constant  Value=[0,0,0;0,0,0]
  FakeStrideTime1 : Constant
  FakeStrideTime_s : Outport
  FakeTime : Outport  Port=2
  wires:
  FakeCoefsTime/1 -> Bus Creator13/2  "coefs"
  FakeBreaksTime/1 -> Bus Creator13/1  "breaks"
  Bus Creator13/1 -> FakeTime/1  "Time"
  FakeStrideTime1/1 -> FakeStrideTime_s/1

== system LopesDevelopmentLibrary/GaitGenerationExtra/CalculateBreaksCoefs/Calculate/LeftAnkleZ1 ==
  note: Maximum of 15 cm extra circumduction
  parameters : Inport
  WeightShift_StepWidth_pct : Inport  Port=2
  Circumduction_CircumductionLeft_pct : Inport  Port=3
  AddToMatrixElement : LopesDevelopmentLibrary/Various/AddToMatrixElement  row=3  col=2  minimum=-inf  maximum=inf
  AssignMatrixElement : LopesDevelopmentLibrary/Various/AssignMatrixElement  row=3  col=2  minimum=-inf  maximum=inf
  Bias : Bias  Bias=1
  CircumductionGain : Gain  Gain=0.01*(-0.15)
  Gain2 : Gain  Gain=0.01
  K1toK3 : dspmtrx3/Submatrix  RowSpan=All rows  RowStartMode=Index  RowStartIndex=row  RowEndMode=Index  RowEndIndex=1  ColSpan=One column  ColStartMode=Index  ColStartIndex=2  ColEndMode=Last  ColEndIndex=1
  MinMax : MinMax
  MultiplyMatrixElement : LopesDevelopmentLibrary/Various/MultiplyMatrixElement  row=1  col=2  minimum=-inf  maximum=inf
  MultiplyMatrixElement1 : LopesDevelopmentLibrary/Various/MultiplyMatrixElement  row=2  col=2  minimum=-inf  maximum=inf
  RegressionData : Constant  Value=LopesParams.GaitData.LAnkleZ
  RegressionData2KeyEvents : LopesDevelopmentLibrary/BlocksForInternalUse/GaitGeneration/RegressionData2KeyEvents
  KeyEvents : Outport
  wires:
  RegressionData2KeyEvents/1 -> MultiplyMatrixElement/1
  RegressionData/1 -> RegressionData2KeyEvents/1
  parameters/1 -> RegressionData2KeyEvents/2
  WeightShift_StepWidth_pct/1 -> Gain2/1
  Gain2/1 -> Bias/1
  Bias/1 -> MultiplyMatrixElement/2, MultiplyMatrixElement1/2
  AddToMatrixElement/1 -> KeyEvents/1
  MultiplyMatrixElement/1 -> MultiplyMatrixElement1/1
  MultiplyMatrixElement1/1 -> K1toK3/1, AssignMatrixElement/1
  K1toK3/1 -> MinMax/1
  MinMax/1 -> AssignMatrixElement/2
  AssignMatrixElement/1 -> AddToMatrixElement/1
  Circumduction_CircumductionLeft_pct/1 -> CircumductionGain/1
  CircumductionGain/1 -> AddToMatrixElement/2

== system LopesDevelopmentLibrary/GaitGenerationExtra/CalculateBreaksCoefs/Calculate/LeftHipFlexion1 ==
  parameters : Inport
  HipExtensionOffset_pct : Inport  Port=2
  Steplength_Length_pct : Inport  Port=3
  SteplengthOtherLeg_Length_pct : Inport  Port=4
  StepHeight_KneeFlexion_pct : Inport  Port=5
  AddToMatrixColumn : LopesDevelopmentLibrary/Various/AddToMatrixColumn  col=2  minimum=-inf  maximum=inf
  Bias : Bias  Bias=100
  Bias1 : Bias  Bias=100
  Gain1 : Gain  Gain=1/100
  Gain2 : Gain  Gain=1/100
  Gain3 : Gain  Gain=0.01* d2r(2.5)
  Gain4 : Gain  Gain=0.01* d2r(5)
  GainHipExtensionOffset : Gain  Gain=-0.01* d2r(10)
  KneeFlexionStepheight : LopesDevelopmentLibrary/Various/AddToMatrixElement  row=5  col=2  minimum=0  maximum=d2r(90)
  KneeFlexionStepheight1 : LopesDevelopmentLibrary/Various/AddToMatrixElement  row=6  col=2  minimum=0  maximum=d2r(90)
  MultiplyMatrixElement : LopesDevelopmentLibrary/Various/MultiplyMatrixElement  row=6  col=2  minimum=-inf  maximum=inf
  MultiplyMatrixElement1 : LopesDevelopmentLibrary/Various/MultiplyMatrixElement  row=4  col=2  minimum=-inf  maximum=inf
  MultiplyMatrixElement2 : LopesDevelopmentLibrary/Various/MultiplyMatrixElement  row=1  col=2  minimum=-inf  maximum=inf
  MultiplyMatrixElement3 : LopesDevelopmentLibrary/Various/MultiplyMatrixElement  row=2  col=2  minimum=-inf  maximum=inf
  RatioFlexionExtension : Gain
  RegressionData : Constant  Value=LopesParams.GaitData.LHF
  RegressionData2KeyEvents : LopesDevelopmentLibrary/BlocksForInternalUse/GaitGeneration/RegressionData2KeyEvents
  KeyEvents : Outport
  wires:
  MultiplyMatrixElement1/1 -> KeyEvents/1
  AddToMatrixColumn/1 -> MultiplyMatrixElement/1
  Gain2/1 -> MultiplyMatrixElement1/2
  Steplength_Length_pct/1 -> Bias/1
  Bias/1 -> Gain1/1
  Gain1/1 -> MultiplyMatrixElement3/2, MultiplyMatrixElement2/2, MultiplyMatrixElement/2
  Bias1/1 -> Gain2/1
  SteplengthOtherLeg_Length_pct/1 -> RatioFlexionExtension/1
  RegressionData/1 -> RegressionData2KeyEvents/1
  parameters/1 -> RegressionData2KeyEvents/2
  KneeFlexionStepheight/1 -> KneeFlexionStepheight1/1
  RegressionData2KeyEvents/1 -> KneeFlexionStepheight/1
  Gain3/1 -> KneeFlexionStepheight/2
  Gain4/1 -> KneeFlexionStepheight1/2
  StepHeight_KneeFlexion_pct/1 -> Gain4/1, Gain3/1
  HipExtensionOffset_pct/1 -> GainHipExtensionOffset/1
  KneeFlexionStepheight1/1 -> AddToMatrixColumn/1
  GainHipExtensionOffset/1 -> AddToMatrixColumn/2
  RatioFlexionExtension/1 -> Bias1/1
  MultiplyMatrixElement/1 -> MultiplyMatrixElement2/1
  MultiplyMatrixElement2/1 -> MultiplyMatrixElement3/1
  MultiplyMatrixElement3/1 -> MultiplyMatrixElement1/1

== system LopesDevelopmentLibrary/GaitGenerationExtra/CalculateBreaksCoefs/Calculate/LeftKneeFlexion1 ==
  parameters : Inport
  StepHeight_KneeFlexion_pct : Inport  Port=2
  Prepositioning_KneeFlexion_pct : Inport  Port=3
  StabilityStance_Kneeflexion_pct : Inport  Port=4
  StepLength_pct : Inport  Port=5
  Constant : Constant  Value=-inf
  Gain1 : Gain  Gain=0.01* d2r(5)
  Gain2 : Gain  Gain=0.01* d2r(10)
  Gain3 : Gain  Gain=0.01* d2r(5)
  Gain4 : Gain  Gain=0.01* d2r(20)
  Gain5 : Gain  Gain=-0.01/3
  KneeFlexionPrepositioning : LopesDevelopmentLibrary/Various/AddToMatrixElement  row=1  col=2  minimum=0  maximum=d2r(90)
  KneefFlexionStepheigh : LopesDevelopmentLibrary/Various/AddToMatrixElement  row=5  col=2  minimum=0  maximum=d2r(90)
  KneefFlexionStepheigh1 : LopesDevelopmentLibrary/Various/AddToMatrixElement  row=6  col=2  minimum=0  maximum=d2r(90)
  KneeflexionStance : LopesDevelopmentLibrary/Various/AddToMatrixElement  row=2  col=2  minimum=0  maximum=d2r(90)
  RatioKey6toKey1 : Gain  Gain=1/2
  RegressionData : Constant  Value=LopesParams.GaitData.LKF
  RegressionData2KeyEvents : LopesDevelopmentLibrary/BlocksForInternalUse/GaitGeneration/RegressionData2KeyEvents
  Saturation : Saturate  UpperLimit=0  LowerLimit=-inf
  Saturation Dynamic : simulink/Discontinuities/Saturation Dynamic  OutMin=[]  OutMax=[]  OutDataTypeStr=Inherit: Same as second input  OutDataType=fixdt(1, 16)  OutScaling=2^-10  DoSatur=off
  SelectorK1 : Selector  NumberOfDimensions=2  InputPortWidth=3  IndexOptions=Index vector (dialog),Index vector (dialog)  Indices=1,2  OutputSizes=1,1
  SelectorK2 : Selector  NumberOfDimensions=2  InputPortWidth=3  IndexOptions=Index vector (dialog),Index vector (dialog)  Indices=2,2  OutputSizes=1,1
  Steplength1 : LopesDevelopmentLibrary/Various/AddToMatrixElement  row=1  col=2  minimum=0  maximum=d2r(90)
  Steplength2 : LopesDevelopmentLibrary/Various/AddToMatrixElement  row=6  col=2  minimum=0  maximum=d2r(90)
  Sum : Sum  Inputs=++|
  Sum1 : Sum  Inputs=-+|
  KeyEvents : Outport
  wires:
  Gain1/1 -> KneeFlexionPrepositioning/2
  StabilityStance_Kneeflexion_pct/1 -> Gain3/1
  Prepositioning_KneeFlexion_pct/1 -> Gain1/1
  RegressionData/1 -> RegressionData2KeyEvents/1
  parameters/1 -> RegressionData2KeyEvents/2
  KneeFlexionPrepositioning/1 -> KneeflexionStance/1
  RegressionData2KeyEvents/1 -> KneefFlexionStepheigh/1
  KneefFlexionStepheigh/1 -> KneefFlexionStepheigh1/1
  StepHeight_KneeFlexion_pct/1 -> Gain4/1, Gain2/1
  Gain2/1 -> KneefFlexionStepheigh/2
  Gain3/1 -> KneeflexionStance/2
  KneefFlexionStepheigh1/1 -> KneeFlexionPrepositioning/1
  Gain4/1 -> KneefFlexionStepheigh1/2
  StepLength_pct/1 -> Saturation/1
  Steplength1/1 -> Steplength2/1
  Steplength2/1 -> KeyEvents/1
  KneeflexionStance/1 -> SelectorK1/1, SelectorK2/1, Steplength1/1
  RatioKey6toKey1/1 -> Steplength2/2
  SelectorK2/1 -> Saturation Dynamic/1
  Constant/1 -> Saturation Dynamic/3
  SelectorK1/1 -> Sum1/1, Sum/1
  Gain5/1 -> Sum/2
  Sum/1 -> Saturation Dynamic/2
  Sum1/1 -> RatioKey6toKey1/1, Steplength1/2
  Saturation Dynamic/1 -> Sum1/2
  Saturation/1 -> Gain5/1

== system LopesDevelopmentLibrary/GaitGenerationExtra/CalculateBreaksCoefs/Calculate/PelvisAxialRotation1 ==
  parameters : Inport
  RegressionData : Constant  Value=LopesParams.GaitData.PAX
  RegressionData2KeyEvents : LopesDevelopmentLibrary/BlocksForInternalUse/GaitGeneration/RegressionData2KeyEvents
  KeyEvents : Outport
  wires:
  parameters/1 -> RegressionData2KeyEvents/2
  RegressionData/1 -> RegressionData2KeyEvents/1
  RegressionData2KeyEvents/1 -> KeyEvents/1

== system LopesDevelopmentLibrary/GaitGenerationExtra/CalculateBreaksCoefs/Calculate/PelvisObliquity1 ==
  parameters : Inport
  RegressionData : Constant  Value=LopesParams.GaitData.POB
  RegressionData2KeyEvents : LopesDevelopmentLibrary/BlocksForInternalUse/GaitGeneration/RegressionData2KeyEvents
  KeyEvents : Outport
  wires:
  RegressionData2KeyEvents/1 -> KeyEvents/1
  RegressionData/1 -> RegressionData2KeyEvents/1
  parameters/1 -> RegressionData2KeyEvents/2

== system LopesDevelopmentLibrary/GaitGenerationExtra/CalculateBreaksCoefs/Calculate/PelvisTX1 ==
  parameters : Inport
  RegressionData : Constant  Value=LopesParams.GaitData.PX
  RegressionData2KeyEvents : LopesDevelopmentLibrary/BlocksForInternalUse/GaitGeneration/RegressionData2KeyEvents
  KeyEvents : Outport
  wires:
  RegressionData2KeyEvents/1 -> KeyEvents/1
  RegressionData/1 -> RegressionData2KeyEvents/1
  parameters/1 -> RegressionData2KeyEvents/2

== system LopesDevelopmentLibrary/GaitGenerationExtra/CalculateBreaksCoefs/Calculate/PelvisTY1 ==
  parameters : Inport
  RegressionData : Constant  Value=LopesParams.GaitData.PY
  RegressionData2KeyEvents : LopesDevelopmentLibrary/BlocksForInternalUse/GaitGeneration/RegressionData2KeyEvents
  KeyEvents : Outport
  wires:
  RegressionData2KeyEvents/1 -> KeyEvents/1
  RegressionData/1 -> RegressionData2KeyEvents/1
  parameters/1 -> RegressionData2KeyEvents/2

== system LopesDevelopmentLibrary/GaitGenerationExtra/CalculateBreaksCoefs/Calculate/PelvisTZ1 ==
  Parameters : Inport
  WeightShift_AmplitudeLeft_pct : Inport  Port=2
  WeightShift_AmplitudeRight_pct : Inport  Port=3
  WeightShift_Timing_pct : Inport  Port=4
  WeightShift_DurationLeft_pct : Inport  Port=5
  WeightShift_DurationRight_pct : Inport  Port=6
  AdjustAmplitude : Subsystem
  AdjustDurationLeft : Subsystem  mask{keyEventsToAffect=[1,2], keyEventBeforeAffected=6}
      mask prompts: keyEventsToAffect "Affect which key events (give two)"; keyEventBeforeAffected "Index of key event just before affected ones"
  AdjustDurationRight : Subsystem  mask{keyEventsToAffect=[4,5], keyEventBeforeAffected=3}
      mask prompts: keyEventsToAffect "Affect which key events (give two)"; keyEventBeforeAffected "Index of key event just before affected ones"
  AdjustTiming : LopesDevelopmentLibrary/Various/AddToMatrixColumn  col=1  minimum=-inf  maximum=inf
  Bias : Bias  Bias=1
  Bias1 : Bias  Bias=1
  Gain1 : Gain  Gain=0.01
  Gain2 : Gain  Gain=0.01
  RegressionData : Constant  Value=LopesParams.GaitData.PZ
  RegressionData2KeyEvents : LopesDevelopmentLibrary/BlocksForInternalUse/GaitGeneration/RegressionData2KeyEvents
  Saturation : Saturate  UpperLimit=2  LowerLimit=0
  Saturation1 : Saturate  UpperLimit=2  LowerLimit=0
  KeyEvents : Outport
  wires:
  Bias/1 -> Saturation/1
  RegressionData/1 -> RegressionData2KeyEvents/1
  WeightShift_Timing_pct/1 -> AdjustTiming/2
  WeightShift_DurationLeft_pct/1 -> AdjustDurationLeft/2(V)
  WeightShift_AmplitudeLeft_pct/1 -> Gain2/1
  AdjustAmplitude/1(Y) -> AdjustDurationLeft/1(M)
  AdjustTiming/1 -> KeyEvents/1
  Gain2/1 -> Bias/1
  Parameters/1 -> RegressionData2KeyEvents/2
  RegressionData2KeyEvents/1 -> AdjustAmplitude/1(M)
  Saturation/1 -> AdjustAmplitude/2(V_left)
  AdjustDurationRight/1(Y) -> AdjustTiming/1
  AdjustDurationLeft/1(Y) -> AdjustDurationRight/1(M)
  WeightShift_DurationRight_pct/1 -> AdjustDurationRight/2(V)
  Bias1/1 -> Saturation1/1
  Gain1/1 -> Bias1/1
  WeightShift_AmplitudeRight_pct/1 -> Gain1/1
  Saturation1/1 -> AdjustAmplitude/3(V_right)

== system LopesDevelopmentLibrary/GaitGenerationExtra/CalculateBreaksCoefs/Calculate/RightAnkleZ1 ==
  note: Maximum of 15 cm extra circumduction
  parameters : Inport
  WeightShift_StepWidth_pct : Inport  Port=2
  Circumduction_CircumductionRight_pct : Inport  Port=3
  AddToMatrixElement : LopesDevelopmentLibrary/Various/AddToMatrixElement  row=3  col=2  minimum=-inf  maximum=inf
  AssignMatrixElement : LopesDevelopmentLibrary/Various/AssignMatrixElement  row=3  col=2  minimum=-inf  maximum=inf
  Bias : Bias  Bias=1
  CircumductionGain : Gain  Gain=0.01*(0.15)
  Gain2 : Gain  Gain=0.01
  K1toK3 : dspmtrx3/Submatrix  RowSpan=All rows  RowStartMode=Index  RowStartIndex=row  RowEndMode=Index  RowEndIndex=1  ColSpan=One column  ColStartMode=Index  ColStartIndex=2  ColEndMode=Last  ColEndIndex=1
  MinMax : MinMax  Function=max
  MultiplyMatrixElement : LopesDevelopmentLibrary/Various/MultiplyMatrixElement  row=1  col=2  minimum=-inf  maximum=inf
  MultiplyMatrixElement1 : LopesDevelopmentLibrary/Various/MultiplyMatrixElement  row=2  col=2  minimum=-inf  maximum=inf
  RegressionData : Constant  Value=LopesParams.GaitData.RAnkleZ
  RegressionData2KeyEvents : LopesDevelopmentLibrary/BlocksForInternalUse/GaitGeneration/RegressionData2KeyEvents
  KeyEvents : Outport
  wires:
  CircumductionGain/1 -> AddToMatrixElement/2
  Circumduction_CircumductionRight_pct/1 -> CircumductionGain/1
  AssignMatrixElement/1 -> AddToMatrixElement/1
  MinMax/1 -> AssignMatrixElement/2
  K1toK3/1 -> MinMax/1
  MultiplyMatrixElement1/1 -> AssignMatrixElement/1, K1toK3/1
  MultiplyMatrixElement/1 -> MultiplyMatrixElement1/1
  AddToMatrixElement/1 -> KeyEvents/1
  Bias/1 -> MultiplyMatrixElement1/2, MultiplyMatrixElement/2
  Gain2/1 -> Bias/1
  WeightShift_StepWidth_pct/1 -> Gain2/1
  parameters/1 -> RegressionData2KeyEvents/2
  RegressionData/1 -> RegressionData2KeyEvents/1
  RegressionData2KeyEvents/1 -> MultiplyMatrixElement/1
